simulink model "Part8_realtime"  (R2024b)
settings: Solver=ode5  StartTime=0.0  StopTime=5  FixedStep=0.001  RelTol=1e-3
values from neighbouring files (symbols this model uses):
  A = [0, 1; 0, -1/Tm]    [DesignPart567.m]    (also in DesignPart8.m; DesignPart9Sine.m; DesignPart9Step.m = [0, 1; 0, a22]; Init.m = [0, 1;0, -1/Tm])
  B = [0, km/(gbox.N*Tm)]'    [DesignPart567.m]    (also in DesignPart8.m; DesignPart9Sine.m; DesignPart9Step.m = [0, b2]'; Init.m = [0; drv.dcgain*mot.Kt/(gbox.N1*mot.Req*Jeq)])
  C = [1, 0]    [DesignPart567.m]    (also in DesignPart8.m; DesignPart9Sine.m; DesignPart9Step.m; Init.m)
  Cr = [90, 0]    [DesignPart567.m]    (also in DesignPart8.m = 90)
  delta_est = 1/sqrt(2)    [DesignPart9Step.m]    (also in Init.m)
  K = real(K)    [DesignPart567.m]    (also in DesignPart8.m; DesignPart9Sine.m; DesignPart9Step.m = place(  A,   B, CtrlPoles); Init.m = acker(A,B,poles))
  wc = 2*pi*50    (= 314.159265359)    [DesignPart9Step.m]    (also in Init.m; State_space_1324.m)
undefined symbols (not defined in the file or in its folder): National_Instruments, PCI, sens
libraries: simulink_extras x3, sldrtlib x3
settings Model: SimulationMode=external  ExtModeTrigDuration=1000001  Creator=galeazzolu  LastModifiedBy=galeazzolu
settings DataIOCC: ReturnWorkspaceOutputs=off
settings HardwareCC: ProdBitPerLong=64  ProdHWDeviceType=Intel->x86-64 (Linux 64)
settings RTWCC: Description=Simulink Desktop Real-Time  SystemTargetFile=sldrt.tlc  TemplateMakefile=sldrt.tmf  RTWCompilerOptimization=on
settings CodeAppCC: MaxIdLength=95
settings SimulinkDesktopRealTimeCC: TargetLibSuffix=_sldrt.a  TargetPreCompLibLocation=C:\Program Files\MATLAB\R2024b\toolbox\sldrt\lib\win64  ParMdlRefBuildCompliant=on

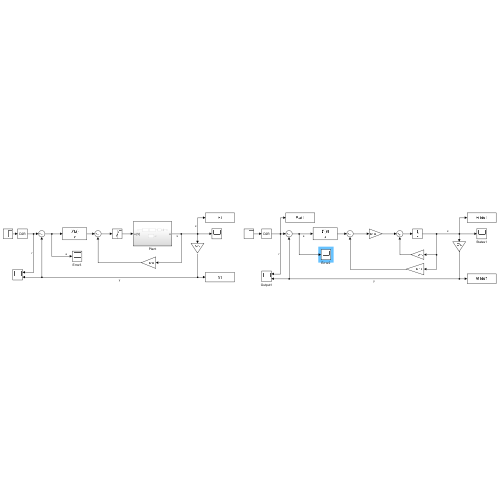
[thumbnail: Simulink's stored preview of the top-level diagram]
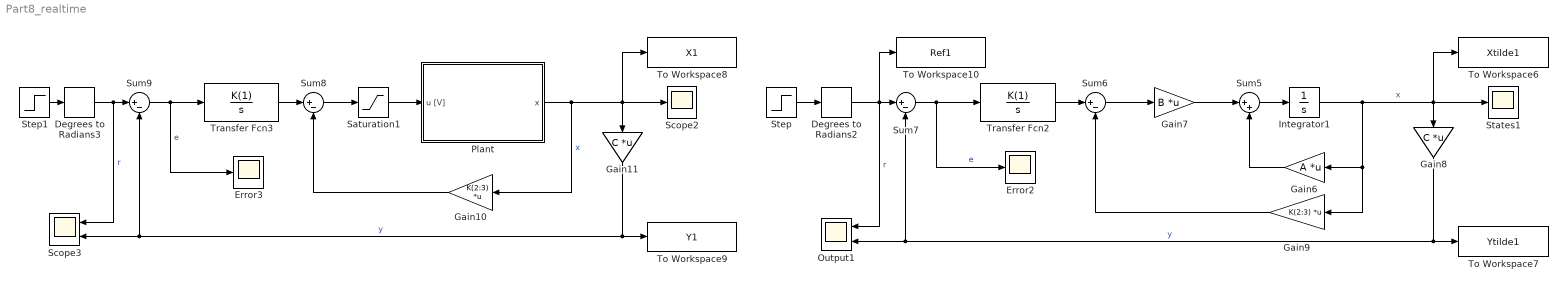
== system Part8_realtime ==
  Degrees to Radians2 : simulink_extras/Transformations/Degrees to Radians
  Degrees to Radians3 : simulink_extras/Transformations/Degrees to Radians
  Error2 : Scope
  Error3 : Scope
  Gain10 : Gain  Gain=K(2:3)  Multiplication=Matrix(K*u)
  Gain11 : Gain  Gain=C  Multiplication=Matrix(K*u)
  Gain6 : Gain  Gain=A  Multiplication=Matrix(K*u)
  Gain7 : Gain  Gain=B  Multiplication=Matrix(K*u)
  Gain8 : Gain  Gain=C  Multiplication=Matrix(K*u)
  Gain9 : Gain  Gain=K(2:3)  Multiplication=Matrix(K*u)
  Integrator1 : Integrator  InitialCondition=rand(2, 1)
  Output1 : Scope  NumInputPorts=2
  Plant : Subsystem
  Saturation1 : Saturate  UpperLimit=10  LowerLimit=-10
  Scope2 : Scope
  Scope3 : Scope  NumInputPorts=2
  States1 : Scope
  Step : Step  After=Cr  SampleTime=0
  Step1 : Step  After=Cr  SampleTime=0
  Sum5 : Sum  Inputs=|++
  Sum{6..9} (4 alike) : Sum  Inputs=|+-
  To Workspace10 : ToWorkspace  VariableName=Ref1  SaveFormat=Timeseries  SampleTime=-1
  To Workspace6 : ToWorkspace  VariableName=Xtilde1  SaveFormat=Timeseries  SampleTime=-1
  To Workspace7 : ToWorkspace  VariableName=Ytilde1  SaveFormat=Timeseries  SampleTime=-1
  To Workspace8 : ToWorkspace  VariableName=X1  SaveFormat=Timeseries  SampleTime=-1
  To Workspace9 : ToWorkspace  VariableName=Y1  SaveFormat=Timeseries  SampleTime=-1
  Transfer Fcn2 : TransferFcn  Numerator=K(1)  Denominator=[1 0]
  Transfer Fcn3 : TransferFcn  Numerator=K(1)  Denominator=[1 0]
  wires:
  Gain8/1 -> To Workspace7/1, Sum7/2, Output1/2  "y"
  Saturation1/1 -> Plant/1(u [V])
  Gain9/1 -> Sum6/2
  Integrator1/1 -> Gain6/1, Gain9/1, To Workspace6/1, Gain8/1, States1/1  "x"
  Degrees to Radians2/1 -> To Workspace10/1, Output1/1, Sum7/1  "r"
  Step/1 -> Degrees to Radians2/1
  Gain6/1 -> Sum5/2
  Sum5/1 -> Integrator1/1
  Sum9/1 -> Error3/1, Transfer Fcn3/1  "e"
  Gain10/1 -> Sum8/2
  Gain7/1 -> Sum5/1
  Plant/1(x) -> To Workspace8/1, Gain11/1, Scope2/1, Gain10/1  "x"
  Sum6/1 -> Gain7/1
  Transfer Fcn2/1 -> Sum6/1
  Sum7/1 -> Error2/1, Transfer Fcn2/1  "e"
  Degrees to Radians3/1 -> Scope3/1, Sum9/1  "r"
  Gain11/1 -> To Workspace9/1, Sum9/2, Scope3/2  "y"
  Transfer Fcn3/1 -> Sum8/1
  Step1/1 -> Degrees to Radians3/1
  Sum8/1 -> Saturation1/1

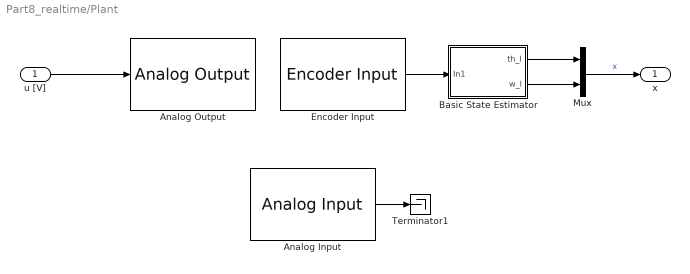
== system Part8_realtime/Plant ==
  u [V] : Inport
  Analog Input : sldrtlib/Analog Input  SampleTime=-1  MaxMissedTicks=10  ShowMissedTicks=off  YieldWhenWaiting=off  DrvName=National_Instruments/PCI-6221  DrvAddress=4294967295  DrvOptions=[0 0 0 2 0]  Channels=[1,2]  RangeMode=1  VoltRange=1  DataType=1
      settings: AttributesFormatString=National Instruments\nPCI-6221 [auto]
  Analog Output : sldrtlib/Analog Output  SampleTime=-1  MaxMissedTicks=10  ShowMissedTicks=off  YieldWhenWaiting=off  DrvName=National_Instruments/PCI-6221  DrvAddress=4294967295  DrvOptions=[0 0 0 2 0]  Channels=1  RangeMode=1  VoltRange=1  InitialValue=0  FinalValue=0
      settings: AttributesFormatString=National Instruments\nPCI-6221 [auto]
  Basic State Estimator : Subsystem
  Encoder Input : sldrtlib/Encoder Input  SampleTime=-1  MaxMissedTicks=10  ShowMissedTicks=off  YieldWhenWaiting=off  DrvName=National_Instruments/PCI-6221  DrvAddress=4294967295  DrvOptions=[0 0 0 2 0]  Channels=1  QuadMode=3  IndexPulse=1  InputFilter=Inf  DataType=1
      settings: AttributesFormatString=National Instruments\nPCI-6221 [auto]
  Mux : Mux  Inputs=2
  Terminator1 : Terminator
  x : Outport
  wires:
  u [V]/1 -> Analog Output/1
  Encoder Input/1 -> Basic State Estimator/1(In1)
  Mux/1 -> x/1  "x"
  Basic State Estimator/1(th_l) -> Mux/1
  Basic State Estimator/2(w_l) -> Mux/2
  Analog Input/1 -> Terminator1/1

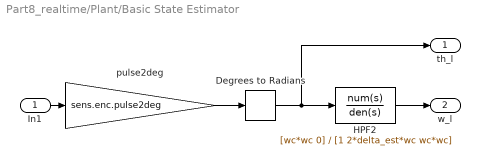
== system Part8_realtime/Plant/Basic State Estimator ==
  In1 : Inport
  Degrees to Radians : simulink_extras/Transformations/Degrees to Radians
  HPF2 : TransferFcn  Numerator=[wc*wc 0]  Denominator=[1 2*delta_est*wc wc*wc]
  pulse2deg : Gain  Gain=sens.enc.pulse2deg
  th_l : Outport
  w_l : Outport  Port=2
  wires:
  pulse2deg/1 -> Degrees to Radians/1
  In1/1 -> pulse2deg/1
  HPF2/1 -> w_l/1
  Degrees to Radians/1 -> th_l/1, HPF2/1
